simulink library "PHIL_lib"  (Simulink 8.1)
settings: Solver=ode45  StartTime=0.0  StopTime=10.0  RelTol=1e-3
values from neighbouring files (symbols this model uses):
  Ts = 100E-6    (= 0.0001)    [BANSHEE_init.m]
undefined symbols (not defined in the file or in its folder): DiscIntNeverNeededParam, PHIL
libraries: powerlib x8, powerlib_extras x5, rtio_opalrt_ml605ex1 x5, powerlib_meascontrol x4, simulink x2, breaker_lib x1
settings Model: Creator=re25624  LastModifiedBy=MGC4

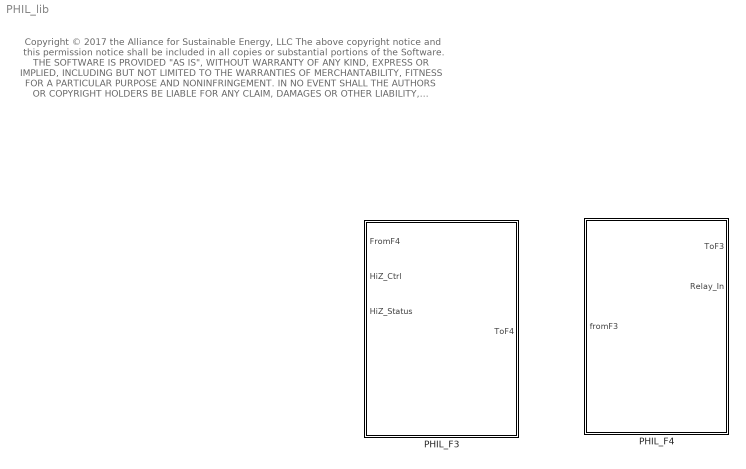
== system PHIL_lib ==
  note: Copyright © 2017 the Alliance for Sustainable Energy, LLC
      |
      | The above copyright notice and this permission notice shall be included in all copies or substantial portions of the Software.
      |
      | THE SOFTWARE IS PROVIDED "AS IS", WITHOUT WARRANTY OF ANY KIND, EXPRESS OR IMPLIED, INCLUDING
      | BUT NOT LIMITED TO THE WARRANTIES OF MERCHANTABILITY, FITNESS FOR A PARTICULAR PURPOSE AND
      | NONINFRINGEMENT. IN NO EVENT SHALL THE AUTHORS OR COPYRIGHT HOLDERS BE LIABLE FOR ANY CLAIM,
      |  DAMAGES OR OTHER LIABILITY, WHETHER IN AN ACTION OF CONTRACT, TORT OR OTHERWISE, ARISING FROM,
      | OUT OF OR IN CONNECTION WITH THE SOFTWARE OR THE USE OR OTHER DEALINGS IN THE SOFTWARE
  PHIL_F3 : Subsystem
  PHIL_F4 : Subsystem

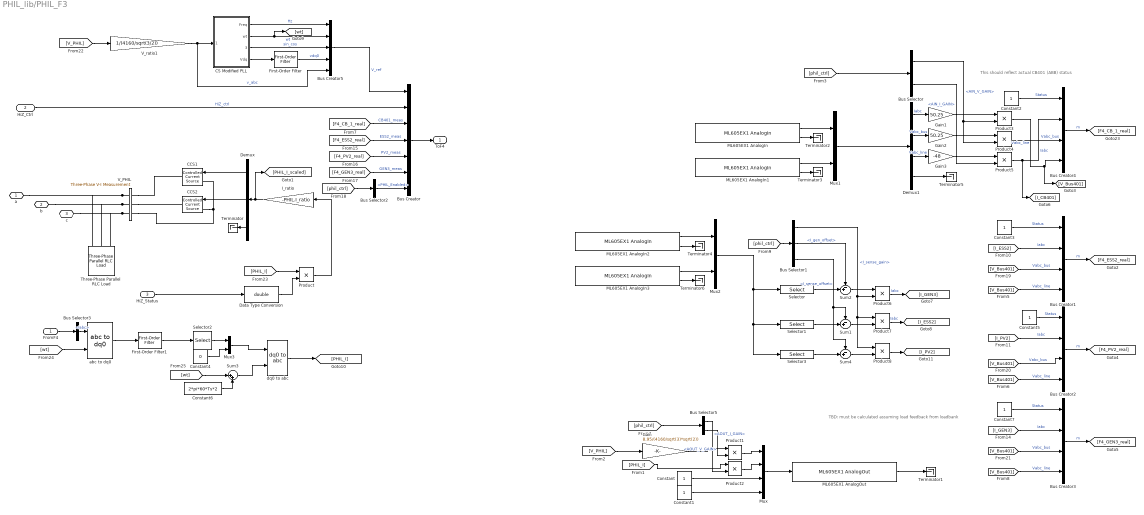
== system PHIL_lib/PHIL_F3 ==
  note: This should reflect actual CB401 (ABB)
      | status
  note: TBD: must be calculated assuming load feedback from loadbank
  FromF4 : Inport
  HiZ_Ctrl : Inport  Port=2
  HiZ_Status : Inport  Port=3
  Bus Creator : BusCreator  Inputs=7
  Bus Creator{1..4} (4 alike) : BusCreator
  Bus Creator5 : BusCreator  Inputs=5
  Bus Selector : BusSelector  OutputSignals=AIN_V_GAIN,AIN_I_GAIN
  Bus Selector1 : BusSelector  OutputSignals=I_sense_gain,I_gen_offset,I_sense_offset
  Bus Selector2 : BusSelector  OutputSignals=PHIL_Enabled
  Bus Selector3 : BusSelector  OutputSignals=Iabc
  Bus Selector5 : BusSelector  OutputSignals=AOUT_I_GAIN,AOUT_V_GAIN
  CCS1 : powerlib/Electrical Sources/Controlled Current Source  Initialize=on  Source_Type=AC  Amplitude=0  Phase=0  Frequency=0  Measurements=None
  CCS2 : powerlib/Electrical Sources/Controlled Current Source  Initialize=on  Source_Type=AC  Amplitude=0  Phase=0  Frequency=0  Measurements=None
  CS Modified PLL : Subsystem  DialogController=POWERSYS.PowerSysDialog  mask(Discrete 3-phase PLL){Flim=[55 66], Par_Init=[0 60], ParK=[ 180 3200 1 ], Ts=Ts, AGC=off}
      mask prompts: Flim "Frequency limits (Hz):"; Par_Init "Initial inputs:[ Phase(degrees)   Frequency(Hz) ]"; ParK "Regulator gains [ Kp  Ki  Kd ]"; Ts "Sample time:"; AGC "Enable Automatic Gain Control"
      mask help:
      | This Phase Locked Loop (PLL) system can be used  to synchronize on a set of variable frequency, three-phase sinusoidal signals. If the Automatic Gain Control is enabled, the input (phase error) of the PLL regulator is scaled according to the input signals magnitude.
      |
      | For optimal performance, the following settings are recommended:
      |   [ Kp Ki  Kd ] = [ 180  3200  1 ]
      |   "Enable Automatic Gain Control" checked
      |
      | Input 1: Vector containing the normalized three-phase signals [Va Vb Vc]
      | Output 1:  Measured frequency (Hz) = w/(2pi)
      | Output 2:  Ramp w.t varying between  0 and 2*pi,
      |      synchronized on zero crossings of the fundamental (positive-sequence) of phase A.
      | Output 3: Vector [sin(wt) cos(wt)]
      mask init:
      | Kp=ParK(1);
      | Ki=ParK(2);
      | if length(ParK)==2
      |     Kd=0;
      | else
      |     Kd=ParK(3);
      | end    
      | Phase_Init=Par_Init(1);
      | Finit=Par_Init(2);
      | %power_initmask();
      settings: OpenFcn=power_openblockproxy();
      mask Display: disp('')
  Constant{,1..3,5,7} (6 alike) : Constant
  Constant4 : Constant  Value=0
  Constant6 : Constant  Value=2*pi*60*Ts*2
  Data Type Conversion : DataTypeConversion  OutDataTypeStr=double
  Demux : Demux  Outputs=3
  Demux1 : Demux  Outputs=[3 3 3 7]
  First-Order Filter : powerlib_meascontrol/Filters/First-Order Filter  FilterType=Lowpass  Tc=10e-3  Ts=Ts  Initialize=on  Vac_Init=[0, 0, 60]  Vdc_Init=0  PlotResponse=off  FreqRange="[0,  200,  1]"
  First-Order Filter1 : powerlib_meascontrol/Filters/First-Order Filter  FilterType=Lowpass  Tc=10e-3  Ts=Ts  Initialize=on  Vac_Init=[0, 0, 60]  Vdc_Init=0  PlotResponse=off  FreqRange="[0,  200,  1]"
  Gain : Gain  Gain=8.95/(4160/sqrt(3)*sqrt(2))
  Gain1 : Gain  Gain=50.25
  Gain2 : Gain  Gain=50.25
  Gain3 : Gain  Gain=-48
  I_ratio : Gain  Gain=-PHIL.I_ratio
  ML605EX1 AnalogIn : rtio_opalrt_ml605ex1/ML605EX1 AnalogIn  CtrlName='ML605EX1 Ctrl'  portNb=1  FcnNos=Slot 1 Module B Subsection 1  size=16  maxcount=8  count=8  numchan=8  sampleTime=0
      settings: AttributesFormatString=%<CtrlName>
  ML605EX1 AnalogIn1 : rtio_opalrt_ml605ex1/ML605EX1 AnalogIn  CtrlName='ML605EX1 Ctrl'  portNb=2  FcnNos=Slot 1 Module B Subsection 2  size=16  maxcount=8  count=8  numchan=8  sampleTime=0
      settings: AttributesFormatString=%<CtrlName>
  ML605EX1 AnalogIn2 : rtio_opalrt_ml605ex1/ML605EX1 AnalogIn  CtrlName='ML605EX1 Ctrl'  portNb=3  FcnNos=Slot 2 Module B Subsection 1  size=16  maxcount=8  count=8  numchan=8  sampleTime=0
      settings: AttributesFormatString=%<CtrlName>
  ML605EX1 AnalogIn3 : rtio_opalrt_ml605ex1/ML605EX1 AnalogIn  CtrlName='ML605EX1 Ctrl'  portNb=4  FcnNos=Slot 2 Module B Subsection 2  size=16  maxcount=8  count=8  numchan=8  sampleTime=0
      settings: AttributesFormatString=%<CtrlName>
  ML605EX1 AnalogOut : rtio_opalrt_ml605ex1/ML605EX1 AnalogOut  CtrlName='ML605EX1 Ctrl'  portNb=1  FcnNos=Slot 1 Module A Subsection 1  size=16  maxcount=8  count=8  numchan=8  israngeinput=off  voltagerange=[-16 ... 16]  slot=0  side=0  mismatch=0  slotside=Slot_1_Module_A
      settings: AttributesFormatString=%<CtrlName>
  Mux : Mux  Inputs=[3 3 1 1]
  Mux1 : Mux  Inputs=2
  Mux2 : Mux  Inputs=2
  Mux3 : Mux  Inputs=2
  Product{,1..8} (9 alike) : Product
  Selector : Selector  InputPortWidth=16  IndexOptions=Index vector (dialog)  Indices=[1 2 4]  OutputSizes=1
  Selector1 : Selector  InputPortWidth=16  IndexOptions=Index vector (dialog)  Indices=[5:7]  OutputSizes=1
  Selector2 : Selector  InputPortWidth=3  IndexOptions=Index vector (dialog)  Indices=[1 2]  OutputSizes=1
  Selector3 : Selector  InputPortWidth=16  IndexOptions=Index vector (dialog)  Indices=[8:10]  OutputSizes=1
  Sum1 : Sum  Inputs=-+|
  Sum2 : Sum  Inputs=-+|
  Sum3 : Sum  Inputs=|++
  Sum4 : Sum  Inputs=-+|
  Terminator{,1..6} (7 alike) : Terminator
  Three-Phase Parallel RLC Load : powerlib/Elements/Three-Phase Parallel RLC Load  LConnTagsString=A|B|C  Configuration=Y (floating)  NominalVoltage=4160  NominalFrequency=60  ActivePower=1e3  InductivePower=0  CapacitivePower=1e3  Measurements=None  LoadType=constant Z
  V_PHIL : powerlib/Measurements/Three-Phase V-I Measurement  VoltageMeasurement=phase-to-ground  SetLabelV=on  LabelV=V_PHIL  Vpu=off  VpuLL=off  CurrentMeasurement=no  SetLabelI=on  LabelI=I_PHIL  Ipu=off  Pbase=100e6  Vbase=500e3  OutputType=Complex  PhasorSimulation=off  PSBequivalent=0
  V_ratio1 : Gain  Gain=1/(4160/sqrt(3/2))
  abc to dq0 : powerlib_meascontrol/Transformations/abc to dq0  Alignment=90 degrees behind phase A axis
  dq0 to abc : powerlib_meascontrol/Transformations/dq0 to abc  Alignment=90 degrees behind phase A axis
  a : PMIOPort  Port=1  Side=Left
  b : PMIOPort  Port=2  Side=Left
  c : PMIOPort  Port=3  Side=Left
  ToF4 : Outport
  wires:
  Bus Selector1/2 -> Sum2/1  "<I_gen_offset>"
  Product8/1 -> [I_PV2]
  Sum4/1 -> Product8/2
  Selector3/1 -> Sum4/2
  FromF4/1 -> Bus Selector3/1
  Bus Selector3/1 -> abc to dq0/1  "<Iabc>"
  dq0 to abc/1 -> [PHIL_I]
  [PHIL_I] -> Product/1
  Sum3/1 -> dq0 to abc/2
  Constant6/1 -> Sum3/2
  [wt] -> Sum3/1
  Constant4/1 -> Mux3/2
  Selector2/1 -> Mux3/1
  Mux3/1 -> dq0 to abc/1
  First-Order Filter1/1 -> Selector2/1
  abc to dq0/1 -> First-Order Filter1/1
  [wt] -> abc to dq0/2
  CS Modified PLL/3(Sin_Cos) -> Bus Creator5/3  "sin_cos"
  CS Modified PLL/1(Freq) -> Bus Creator5/1  "Hz"
  CS Modified PLL/2(wt) -> Bus Creator5/2, [wt]  "wt"
  First-Order Filter/1 -> Bus Creator5/4  "vdq0"
  CS Modified PLL/4(Vdq) -> First-Order Filter/1
  V_ratio1/1 -> CS Modified PLL/1(Vabc(pu)), Bus Creator5/5  "v_abc"
  [V_PHIL] -> V_ratio1/1
  Bus Selector2/1 -> Bus Creator/7  "<PHIL_Enabled>"
  [phil_ctrl] -> Bus Selector2/1
  [F4_GEN3_real] -> Bus Creator/6  "GEN3_meas"
  [F4_PV2_real] -> Bus Creator/5  "PV2_meas"
  [F4_ESS2_real] -> Bus Creator/4  "ESS2_meas"
  Product7/1 -> [I_ESS2]  "Iabc"
  Product6/1 -> [I_GEN3]  "Iabc"
  Bus Selector1/1 -> Product6/2, Product7/1, Product8/1  "<I_sense_gain>"
  Bus Selector1/3 -> Sum1/1, Sum4/1  "<I_sense_offset>"
  [phil_ctrl] -> Bus Selector1/1
  Sum1/1 -> Product7/2
  Sum2/1 -> Product6/1
  [I_GEN3] -> Bus Creator3/2  "Iabc"
  [V_Bus401] -> Bus Creator3/3  "Vabc_bus"
  [V_Bus401] -> Bus Creator3/4  "Vabc_line"
  Constant7/1 -> Bus Creator3/1  "Status"
  Bus Creator3/1 -> [F4_GEN3_real]  "m"
  Selector1/1 -> Sum1/2
  [I_PV2] -> Bus Creator2/2  "Iabc"
  [V_Bus401] -> Bus Creator2/3  "Vabc_bus"
  [V_Bus401] -> Bus Creator2/4  "Vabc_line"
  Constant5/1 -> Bus Creator2/1  "Status"
  Bus Creator2/1 -> [F4_PV2_real]  "m"
  Selector/1 -> Sum2/2
  [I_ESS2] -> Bus Creator1/2  "Iabc"
  [V_Bus401] -> Bus Creator1/3  "Vabc_bus"
  [V_Bus401] -> Bus Creator1/4  "Vabc_line"
  Constant3/1 -> Bus Creator1/1  "Status"
  Bus Creator1/1 -> [F4_ESS2_real]  "m"
  Mux2/1 -> Selector1/1, Selector3/1, Selector/1
  ML605EX1 AnalogIn3/1 -> Mux2/2
  ML605EX1 AnalogIn2/1 -> Mux2/1
  ML605EX1 AnalogIn3/2 -> Terminator6/1
  ML605EX1 AnalogIn2/2 -> Terminator4/1
  [phil_ctrl] -> Bus Selector/1
  Product2/1 -> Mux/2
  Product1/1 -> Mux/1
  Bus Selector5/1 -> Product2/2  "<AOUT_I_GAIN>"
  Bus Selector5/2 -> Product1/2  "<AOUT_V_GAIN>"
  Gain/1 -> Product1/1
  [phil_ctrl] -> Bus Selector5/1
  ML605EX1 AnalogOut/1 -> Terminator1/1
  [PHIL_I] -> Product2/1
  Constant1/1 -> Mux/4
  Constant/1 -> Mux/3
  [V_PHIL] -> Gain/1
  Mux/1 -> ML605EX1 AnalogOut/1
  Gain3/1 -> Product5/1
  Gain2/1 -> Product4/1
  Gain1/1 -> Product3/1
  ML605EX1 AnalogIn1/1 -> Mux1/2
  ML605EX1 AnalogIn1/2 -> Terminator3/1
  ML605EX1 AnalogIn/2 -> Terminator2/1
  ML605EX1 AnalogIn/1 -> Mux1/1
  Mux1/1 -> Demux1/1
  Bus Selector/2 -> Product5/2  "<AIN_I_GAIN>"
  Bus Selector/1 -> Product3/2, Product4/2  "<AIN_V_GAIN>"
  Demux1/3 -> Gain3/1  "Vabc_line"
  Demux1/2 -> Gain2/1  "Vabc_bus"
  Demux1/1 -> Gain1/1  "Iabc"
  Product5/1 -> Bus Creator4/2, [I_CB401]  "Iabc"
  Product4/1 -> Bus Creator4/3  "Vabc_bus"
  Product3/1 -> Bus Creator4/4, [V_Bus401]  "Vabc_line"
  Constant2/1 -> Bus Creator4/1  "Status"
  Bus Creator4/1 -> [F4_CB_1_real]  "m"
  Demux1/4 -> Terminator5/1
  [F4_CB_1_real] -> Bus Creator/3  "CB401_meas"
  Bus Creator/1 -> ToF4/1
  Bus Creator5/1 -> Bus Creator/1  "V_ref"
  HiZ_Ctrl/1 -> Bus Creator/2  "HiZ_ctrl"
  Demux/2 -> CCS2/1
  Demux/1 -> CCS1/1
  I_ratio/1 -> Demux/1, [PHIL_I_scaled]
  Demux/3 -> Terminator/1
  Product/1 -> I_ratio/1
  Data Type Conversion/1 -> Product/2
  HiZ_Status/1 -> Data Type Conversion/1
  connections:
  CCS2/LConn1 -- V_PHIL/RConn3 -- CCS1/LConn1
  V_PHIL/RConn1 -- CCS1/RConn1
  V_PHIL/RConn2 -- CCS2/RConn1
  V_PHIL/LConn3 -- Three-Phase Parallel RLC Load/LConn3 -- c/RConn1
  V_PHIL/LConn2 -- Three-Phase Parallel RLC Load/LConn2 -- b/RConn1
  V_PHIL/LConn1 -- Three-Phase Parallel RLC Load/LConn1 -- a/RConn1

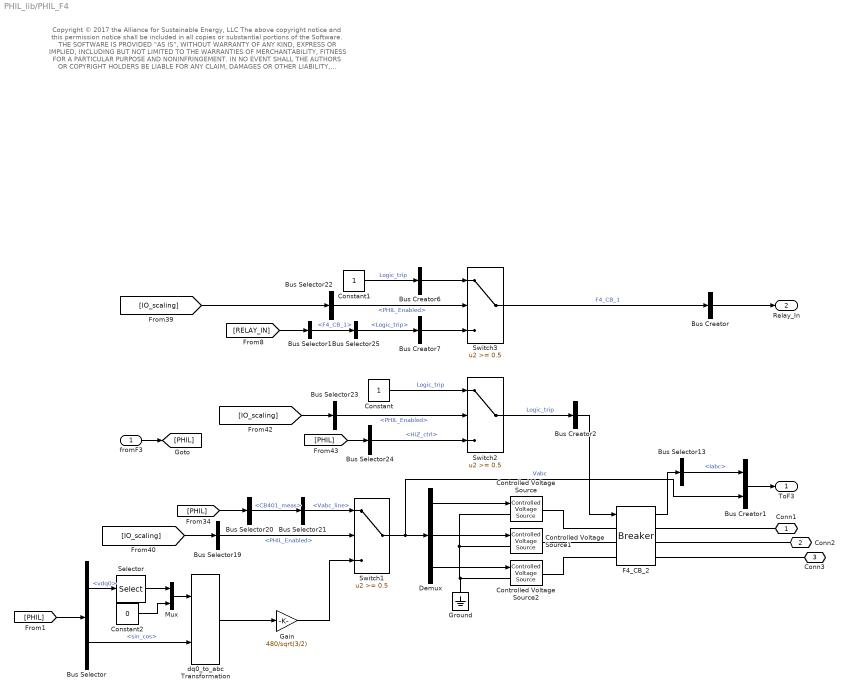
== system PHIL_lib/PHIL_F4 ==
  note: Copyright © 2017 the Alliance for Sustainable Energy, LLC
      |
      | The above copyright notice and this permission notice shall be included in all copies or substantial portions of the Software.
      |
      | THE SOFTWARE IS PROVIDED "AS IS", WITHOUT WARRANTY OF ANY KIND, EXPRESS OR IMPLIED, INCLUDING
      | BUT NOT LIMITED TO THE WARRANTIES OF MERCHANTABILITY, FITNESS FOR A PARTICULAR PURPOSE AND
      | NONINFRINGEMENT. IN NO EVENT SHALL THE AUTHORS OR COPYRIGHT HOLDERS BE LIABLE FOR ANY CLAIM,
      |  DAMAGES OR OTHER LIABILITY, WHETHER IN AN ACTION OF CONTRACT, TORT OR OTHERWISE, ARISING FROM,
      | OUT OF OR IN CONNECTION WITH THE SOFTWARE OR THE USE OR OTHER DEALINGS IN THE SOFTWARE
  fromF3 : Inport
  Bus Creator{,2,6..7} (4 alike) : BusCreator  Inputs=1
  Bus Creator1 : BusCreator  Inputs=2
  Bus Selector : BusSelector  OutputSignals=V_ref.vdq0,V_ref.sin_cos
  Bus Selector1 : BusSelector  OutputSignals=F4_CB_1
  Bus Selector13 : BusSelector  OutputSignals=Iabc
  Bus Selector19 : BusSelector  OutputSignals=PHIL_Enabled
  Bus Selector20 : BusSelector  OutputSignals=CB401_meas
  Bus Selector21 : BusSelector  OutputSignals=Vabc_line
  Bus Selector22 : BusSelector  OutputSignals=PHIL_Enabled
  Bus Selector23 : BusSelector  OutputSignals=PHIL_Enabled
  Bus Selector24 : BusSelector  OutputSignals=HiZ_ctrl
  Bus Selector25 : BusSelector  OutputSignals=Logic_trip
  Constant : Constant
  Constant1 : Constant
  Constant2 : Constant  Value=0
  Controlled Voltage Source : powerlib/Electrical Sources/Controlled Voltage Source  Initialize=on  Source_Type=AC  Amplitude=0  Phase=0  Frequency=0  Measurements=None
  Controlled Voltage Source1 : powerlib/Electrical Sources/Controlled Voltage Source  Initialize=on  Source_Type=AC  Amplitude=0  Phase=0  Frequency=0  Measurements=None
  Controlled Voltage Source2 : powerlib/Electrical Sources/Controlled Voltage Source  Initialize=on  Source_Type=AC  Amplitude=0  Phase=0  Frequency=0  Measurements=None
  Demux : Demux  Outputs=3
  F4_CB_2 : breaker_lib/Breaker  Ts=Ts  mech_delay=cb_mech_delay
  Gain : Gain  Gain=480/sqrt(3/2)
  Ground : powerlib/Elements/Ground  LConnTagsString=a
  Mux : Mux  Inputs=2
  Selector : Selector  InputPortWidth=3  IndexOptions=Index vector (dialog)  Indices=[1 2]  OutputSizes=1
  Switch1 : Switch  Threshold=0.5
  Switch2 : Switch  Threshold=0.5
  Switch3 : Switch  Threshold=0.5
  dq0_to_abc Transformation : powerlib_extras/Measurements/dq0_to_abc Transformation
  Conn1 : PMIOPort  Port=1  Side=Right
  Conn2 : PMIOPort  Port=2  Side=Right
  Conn3 : PMIOPort  Port=3  Side=Right
  ToF3 : Outport
  Relay_In : Outport  Port=2
  wires:
  Switch1/1 -> Demux/1, Bus Creator1/2  "Vabc"
  Bus Creator1/1 -> ToF3/1
  Gain/1 -> Switch1/3
  Bus Selector/2 -> dq0_to_abc Transformation/2  "<sin_cos>"
  Constant2/1 -> Mux/2
  Selector/1 -> Mux/1
  Mux/1 -> dq0_to_abc Transformation/1
  Bus Selector/1 -> Selector/1  "<vdq0>"
  [PHIL] -> Bus Selector/1
  dq0_to_abc Transformation/1 -> Gain/1
  fromF3/1 -> [PHIL]
  Bus Creator2/1 -> F4_CB_2/1
  Bus Creator/1 -> Relay_In/1
  Bus Creator7/1 -> Switch3/3
  Bus Selector25/1 -> Bus Creator7/1  "<Logic_trip>"
  Bus Selector24/1 -> Switch2/3  "<HiZ_ctrl>"
  [PHIL] -> Bus Selector24/1
  Bus Selector23/1 -> Switch2/2  "<PHIL_Enabled>"
  [IO_scaling] -> Bus Selector23/1
  Switch3/1 -> Bus Creator/1  "F4_CB_1"
  Constant1/1 -> Bus Creator6/1  "Logic_trip"
  Bus Creator6/1 -> Switch3/1
  Bus Selector22/1 -> Switch3/2  "<PHIL_Enabled>"
  [IO_scaling] -> Bus Selector22/1
  Switch2/1 -> Bus Creator2/1  "Logic_trip"
  Constant/1 -> Switch2/1  "Logic_trip"
  Bus Selector21/1 -> Switch1/1  "<Vabc_line>"
  [PHIL] -> Bus Selector20/1
  Bus Selector19/1 -> Switch1/2  "<PHIL_Enabled>"
  [IO_scaling] -> Bus Selector19/1
  Bus Selector20/1 -> Bus Selector21/1  "<CB401_meas>"
  Bus Selector13/1 -> Bus Creator1/1  "<Iabc>"
  F4_CB_2/1 -> Bus Selector13/1
  Demux/3 -> Controlled Voltage Source2/1
  Demux/2 -> Controlled Voltage Source1/1
  Demux/1 -> Controlled Voltage Source/1
  Bus Selector1/1 -> Bus Selector25/1  "<F4_CB_1>"
  [RELAY_IN] -> Bus Selector1/1
  connections:
  Controlled Voltage Source2/RConn1 -- F4_CB_2/LConn3
  Controlled Voltage Source1/RConn1 -- F4_CB_2/LConn2
  Controlled Voltage Source/RConn1 -- F4_CB_2/LConn1
  Controlled Voltage Source1/LConn1 -- Controlled Voltage Source/LConn1 -- Controlled Voltage Source2/LConn1 -- Ground/LConn1
  Conn2/RConn1 -- F4_CB_2/RConn2
  Conn1/RConn1 -- F4_CB_2/RConn1
  Conn3/RConn1 -- F4_CB_2/RConn3

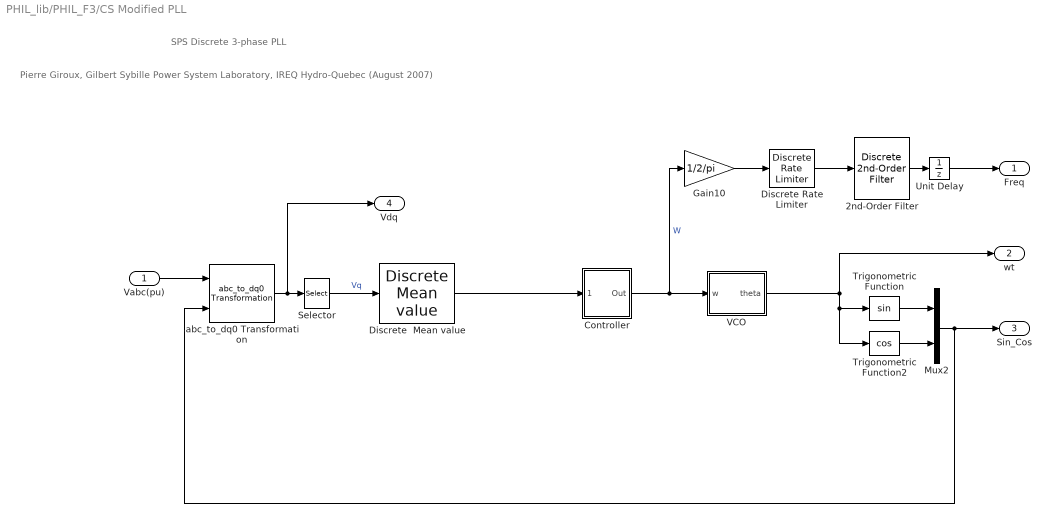
== system PHIL_lib/PHIL_F3/CS Modified PLL ==
  note: Pierre Giroux, Gilbert Sybille
      | Power System Laboratory, IREQ
      | Hydro-Quebec
      | (August 2007)
  note: SPS Discrete 3-phase PLL
  Vabc(pu) : Inport  PortDimensions=3
  2nd-Order Filter : powerlib_extras/Discrete  Control Blocks/Discrete  2nd-Order Filter  FilterType=Lowpass  Fo=25  Zeta=0.707  Ts=Ts  Initialize=on  Vac_Init=[0 0 Finit]  Vdc_Init=Finit  PlotResponse=off  param1=[1 500 0.1]
  Controller : Subsystem  mask(Discrete PID Controller){Kp=Kp, Ki=Ki, Kd=Kd, Par_Limits=[Flim(2) Flim(1)]*2*pi, Init=2*pi*Finit, Ts=Ts}
      mask prompts: Kp "Proportional gain (Kp):"; Ki "Integral gain (Ki):"; Kd "Derivative gain (Kd):"; Par_Limits "Output limits: [ Upper   Lower ]"; Init "Output initial value:"; Ts "Sample time:"
      mask help: This block implements a discrete PID controller.
      mask init:
      | UpperLimit=Par_Limits(1);
      | LowerLimit=Par_Limits(2);
      | power_initmask();
      settings: OpenFcn=power_openblockproxy();
      mask Display: disp('PID');
  Discrete Rate Limiter : powerlib_extras/Discrete  Control Blocks/Discrete Rate Limiter  R=12  F=-12  Vinit=Finit  Ts=Ts
  Discrete  Mean value : powerlib_extras/Discrete Measurements/Discrete  Mean value  Freq=60  Vinit=0  Ts=Ts
  Gain10 : Gain  Gain=1/2/pi  SaturateOnIntegerOverflow=on  OutDataTypeStr=Inherit: Same as input  ParamDataTypeStr=Inherit: Same as input
  Mux2 : Mux  Inputs=2
  Selector : Selector  InputPortWidth=3  IndexOptions=Index vector (dialog)  Indices=2  OutputSizes=1
  Trigonometric Function : Trigonometry
  Trigonometric Function2 : Trigonometry  Operator=cos
  Unit Delay : UnitDelay  InitialCondition=Finit  SampleTime=Ts
  VCO : Subsystem
  abc_to_dq0 Transformation : powerlib_extras/Measurements/abc_to_dq0 Transformation
  Freq : Outport
  wt : Outport  Port=2
  Sin_Cos : Outport  Port=3
  Vdq : Outport  Port=4
  wires:
  Selector/1 -> Discrete  Mean value/1  "Vq"
  2nd-Order Filter/1 -> Unit Delay/1
  Unit Delay/1 -> Freq/1
  Discrete Rate Limiter/1 -> 2nd-Order Filter/1
  Gain10/1 -> Discrete Rate Limiter/1
  Mux2/1 -> Sin_Cos/1, abc_to_dq0 Transformation/2
  Trigonometric Function2/1 -> Mux2/2
  Trigonometric Function/1 -> Mux2/1
  VCO/1(theta) -> wt/1, Trigonometric Function2/1, Trigonometric Function/1
  abc_to_dq0 Transformation/1 -> Selector/1, Vdq/1
  Vabc(pu)/1 -> abc_to_dq0 Transformation/1
  Controller/1(Out) -> Gain10/1, VCO/1(w)  "W"
  Discrete  Mean value/1 -> Controller/1(Error)

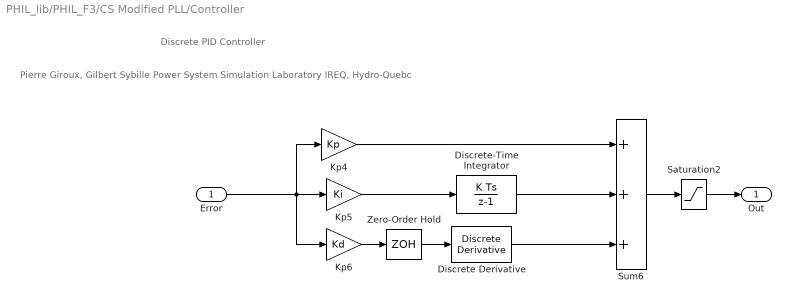
== system PHIL_lib/PHIL_F3/CS Modified PLL/Controller ==
  note: Pierre Giroux, Gilbert Sybille
      | Power System Simulation Laboratory
      | IREQ, Hydro-Quebc
  note: Discrete PID Controller
  Error : Inport
  Discrete Derivative : simulink/Discrete/Discrete Derivative  gainval=1.0  ICPrevScaledInput=0.0  InputProcessing=Inherited  OutMin=[]  OutMax=[]  OutDataType=sfix(16)  OutScaling=2^-10  DoSatur=off
  Discrete-Time Integrator : DiscreteIntegrator  InitialCondition=Init  SampleTime=Ts  LimitOutput=on  UpperSaturationLimit=UpperLimit  LowerSaturationLimit=LowerLimit  ICPrevOutput=DiscIntNeverNeededParam  ICPrevScaledInput=DiscIntNeverNeededParam
  Kp4 : Gain  Gain=Kp  SaturateOnIntegerOverflow=on  OutDataTypeStr=Inherit: Same as input  ParamDataTypeStr=Inherit: Same as input
  Kp5 : Gain  Gain=Ki  SaturateOnIntegerOverflow=on  OutDataTypeStr=Inherit: Same as input  ParamDataTypeStr=Inherit: Same as input
  Kp6 : Gain  Gain=Kd  SaturateOnIntegerOverflow=on  OutDataTypeStr=Inherit: Same as input  ParamDataTypeStr=Inherit: Same as input
  Saturation2 : Saturate  UpperLimit=UpperLimit  LowerLimit=LowerLimit
  Sum6 : Sum  Inputs=+++  SaturateOnIntegerOverflow=on  InputSameDT=on  OutDataTypeStr=Inherit: Same as first input
  Zero-Order Hold : ZeroOrderHold  SampleTime=Ts
  Out : Outport  InitialOutput=0
  wires:
  Error/1 -> Kp4/1, Kp5/1, Kp6/1
  Sum6/1 -> Saturation2/1
  Kp5/1 -> Discrete-Time Integrator/1
  Kp6/1 -> Zero-Order Hold/1
  Kp4/1 -> Sum6/1
  Discrete-Time Integrator/1 -> Sum6/2
  Discrete Derivative/1 -> Sum6/3
  Saturation2/1 -> Out/1
  Zero-Order Hold/1 -> Discrete Derivative/1

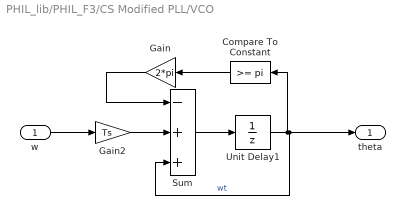
== system PHIL_lib/PHIL_F3/CS Modified PLL/VCO ==
  w : Inport
  Compare To Constant : simulink/Logic and Bit Operations/Compare To Constant  relop=>=  const=pi  OutDataTypeStr=uint8
  Gain : Gain  Gain=2*pi  OutDataTypeStr=double
  Gain2 : Gain  Gain=Ts  SaturateOnIntegerOverflow=on  OutDataTypeStr=Inherit: Same as input  ParamDataTypeStr=Inherit: Same as input
  Sum : Sum  Inputs=-++
  Unit Delay1 : UnitDelay  SampleTime=-1
  theta : Outport
  wires:
  w/1 -> Gain2/1
  Gain/1 -> Sum/1
  Compare To Constant/1 -> Gain/1
  Unit Delay1/1 -> Compare To Constant/1, Sum/3, theta/1  "wt"
  Gain2/1 -> Sum/2
  Sum/1 -> Unit Delay1/1
